simulink model "ctc"  (R2014a)
settings: Solver=ode45  StartTime=0.0  StopTime=10.0  RelTol=1e-3
StopFcn:
  | if(exist('Q'))
  | 
  | pause_time = 0.001;
  | pause_on = 1;
  | 
  | figure(2)
  | h=uicontrol(gcf,'style','pushbutton','String','PLAY','position',[175 5 200 30]);
  | set(h,'callback','if(pause_on == 1); for i=1:size(Q.Data,1); plot(Rob, Q.Data(i,:));pause(pause_time); end; end; if(pause_on == 0); for i=1:size(Q.Data,1) plot(Rob, Q.Data(i,:)); end; end;');
  | 
  | h=uicontrol(gcf,'style','pushbutton','String','make slower','position',[50 5 100 30]);
  | set(h,'callback','pause_time = pause_time*2; if(pause_time>1e-4) pause_on = 1; end');
  | 
  | h=uicontrol(gcf,'style','pushbutton','String','make faster','position',[400 5 100 30]);
  | set(h,'callback','if(pause_time<1e-4) pause_on = 0; else; pause_time = pause_time/2; end ');
  | 
  | set(gcf, 'toolbar', 'figure')
  | 
  | end
undefined symbols (not defined in the file or in its folder): q, qd, qdd
undefined symbols (not defined in the file): perturb, Rob
settings Model: Creator=user  LastModifiedBy=Wolfgang
settings SolverCC: ZeroCrossAlgorithm=Adaptive
settings OptimizationCC: SimCompilerOptimization=On
settings DebuggingCC: UnderspecifiedInitializationDetection=Classic  SolverPrmCheckMsg=none

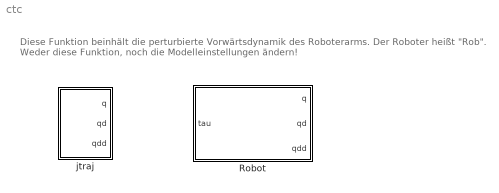
== system ctc ==
  note: Diese Funktion beinhält die perturbierte Vorwärtsdynamik des Roboterarms. Der
      | Roboter heißt "Rob". Weder diese Funktion, noch die Modelleinstellungen ändern!
  Robot : Subsystem  LoadFcn=set_param(gcb,'Name','Robot');  InitFcn=|  mask{robot=perturb(Rob), q0=[0 0 0]}
      | set_param(gcb,'q0','[0 0 0]');
      | set_param(gcb,'Name','Robot');
      | 
      | if(~any(strcmp(who,'Testumgebung')))
      | 
      | if(~strcmp(get_param(gcb,'Robot'),'perturb(Rob)'))
      | set_param(gcb,'Robot','perturb(Rob)');
      | warning('Verändern sie nichts in der Funktion Robot.')
      | end
      | 
      | end
      mask prompts: robot "SerialLink object"; q0 "Initial state"
      mask help: Rigid-body dynamic model of robot.
      mask init:
      | n = robot.n;
      | name = robot.name;
      mask Help: Simulates the forward (direct) rigid-body dynamics of the robot described by the given robot object.
      mask Display:
      | port_label('input', 1, 'tau')
      | port_label('output', 1, 'q')
      | port_label('output', 2, 'qd')
      | port_label('output', 3, 'qdd')
      | text(0.1, 0.9,  robot.name, 'horizontalAlignment', 'left')
  jtraj : Subsystem  mask{q0=0, qf=pi/2, tmax=10}
      mask help: Joint interpolated trajectory.
      mask init:
      | n = length(q0);
      | if length(q0) ~= length(qf) ,
      |  error('q0 and qf must be same length')
      | end
      | t=[0:100]'/100*tmax;
      | [q,qd,qdd] = jtraj(q0, qf, t);
      mask Help:
      | Generate quintic polynomial to move from initial to final joint angles as specified.  Initial and final velocity are assumed to be zero.
      | 
      | Outputs joint angles as well as joint angle rates.
      mask Display:
      | port_label('output', 1, 'q')
      | port_label('output', 2, 'qd')
      | port_label('output', 3, 'qdd')

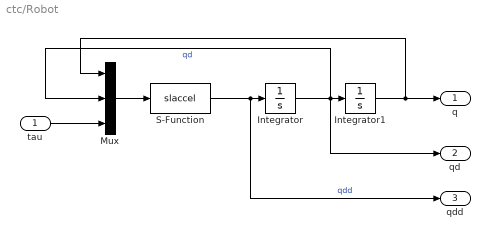
== system ctc/Robot ==
  tau : Inport
  Integrator : Integrator
  Integrator1 : Integrator
  Mux : Mux  Inputs=3
  S-Function : S-Function  FunctionName=slaccel  Parameters=robot  EnableBusSupport=off
  q : Outport
  qd : Outport  Port=2
  qdd : Outport  Port=3
  wires:
  Integrator1/1 -> Mux/1, q/1
  tau/1 -> Mux/3
  Integrator/1 -> Mux/2, Integrator1/1, qd/1  "qd"
  Mux/1 -> S-Function/1
  S-Function/1 -> Integrator/1, qdd/1  "qdd"

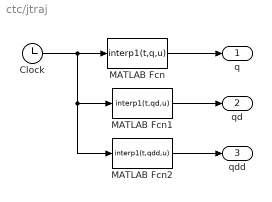
== system ctc/jtraj ==
  Clock : Clock
  MATLAB Fcn : MATLABFcn  MATLABFcn=interp1(t,q,u)  OutputDimensions=n
  MATLAB Fcn1 : MATLABFcn  MATLABFcn=interp1(t,qd,u)  OutputDimensions=n
  MATLAB Fcn2 : MATLABFcn  MATLABFcn=interp1(t,qdd,u)  OutputDimensions=n
  q : Outport
  qd : Outport  Port=2
  qdd : Outport  Port=3
  wires:
  MATLAB Fcn2/1 -> qdd/1
  Clock/1 -> MATLAB Fcn2/1, MATLAB Fcn1/1, MATLAB Fcn/1
  MATLAB Fcn1/1 -> qd/1
  MATLAB Fcn/1 -> q/1
